simulink library "MyMidSideLibrary"  (R2026a)
settings: Solver=VariableStepAuto

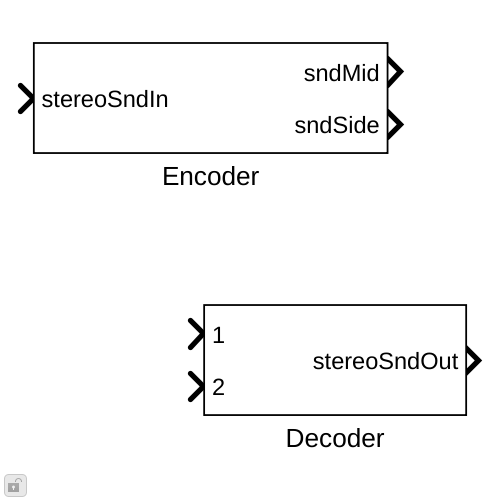
[thumbnail: Simulink's stored preview of the top-level diagram]
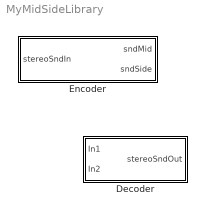
== system MyMidSideLibrary ==
  Decoder : Subsystem
  Encoder : Subsystem

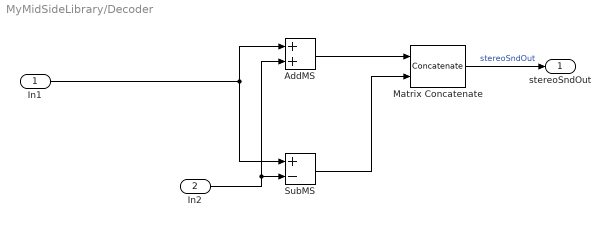
== system MyMidSideLibrary/Decoder ==
  In1 : Inport
  In2 : Inport  Port=2
  AddMS : Sum
  Matrix Concatenate : Concatenate  Mode=Multidimensional array  ConcatenateDimension=2
  SubMS : Sum  Inputs=+-
  stereoSndOut : Outport
  wires:
  In2/1 -> SubMS/2, AddMS/2
  In1/1 -> AddMS/1, SubMS/1
  Matrix Concatenate/1 -> stereoSndOut/1  "stereoSndOut"
  AddMS/1 -> Matrix Concatenate/1
  SubMS/1 -> Matrix Concatenate/2

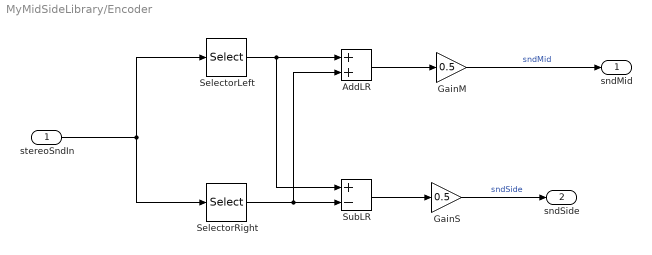
== system MyMidSideLibrary/Encoder ==
  stereoSndIn : Inport
  AddLR : Sum
  GainM : Gain  Gain=0.5
  GainS : Gain  Gain=0.5
  SelectorLeft : Selector  NumberOfDimensions=2  InputPortWidth=3  IndexOptions=Select all,Index vector (dialog)  Indices=[1 3],1  OutputSizes=1,1
  SelectorRight : Selector  NumberOfDimensions=2  InputPortWidth=3  IndexOptions=Select all,Index vector (dialog)  Indices=[1 3],2  OutputSizes=1,1
  SubLR : Sum  Inputs=+-
  sndMid : Outport
  sndSide : Outport  Port=2
  wires:
  SelectorLeft/1 -> SubLR/1, AddLR/1
  SubLR/1 -> GainS/1
  stereoSndIn/1 -> SelectorRight/1, SelectorLeft/1
  GainS/1 -> sndSide/1  "sndSide"
  GainM/1 -> sndMid/1  "sndMid"
  AddLR/1 -> GainM/1
  SelectorRight/1 -> SubLR/2, AddLR/2
